simulink model "sample_hold"  (R2021b)
settings: Solver=VariableStepAuto  StartTime=0.0  StopTime=10.0  RelTol=1e-3
settings Model: Creator=varunsampat  LastModifiedBy=varunsampat

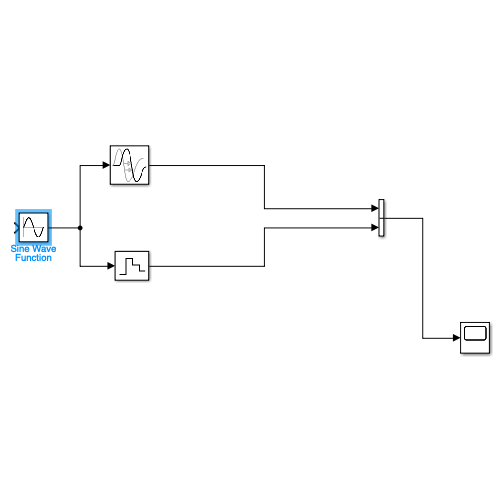
[thumbnail: Simulink's stored preview of the top-level diagram]
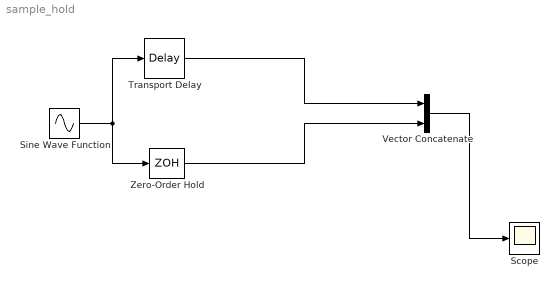
== system sample_hold ==
  Scope : Scope
  Sine Wave Function : Sin  TimeSource=Use external signal  SampleTime=0
  Transport Delay : TransportDelay  DelayTime=0.5
  Vector Concatenate : Concatenate
  Zero-Order Hold : ZeroOrderHold
  wires:
  Sine Wave Function/1 -> Zero-Order Hold/1, Transport Delay/1
  Transport Delay/1 -> Vector Concatenate/1
  Zero-Order Hold/1 -> Vector Concatenate/2
  Vector Concatenate/1 -> Scope/1
